simulink model "ddc_bpm_476_066"  (Simulink 7.8)
settings: Solver=ode45  StartTime=0.0  StopTime=2e-3  RelTol=1e-3
undefined symbols (not defined in the file): decim_factor_poly_35, dt_sim, frev_476, Fs_adc, n_ch, n_ovs, R_fofb, R_sec, R_sec_cfir, R_sec_pfir, xlipgetpartsetting
libraries: xbsIndex_r4 x1136, simulink x7
(part 1 of 10)
settings Model: Creator=lucas.russo  LastModifiedBy=lucas.russo
settings HardwareCC: ProdHWDeviceType=ASIC/FPGA->ASIC/FPGA  TargetIntDivRoundTo=Zero  TargetEndianess=LittleEndian  TargetHWDeviceType=MATLAB Host  ProdEqTarget=off

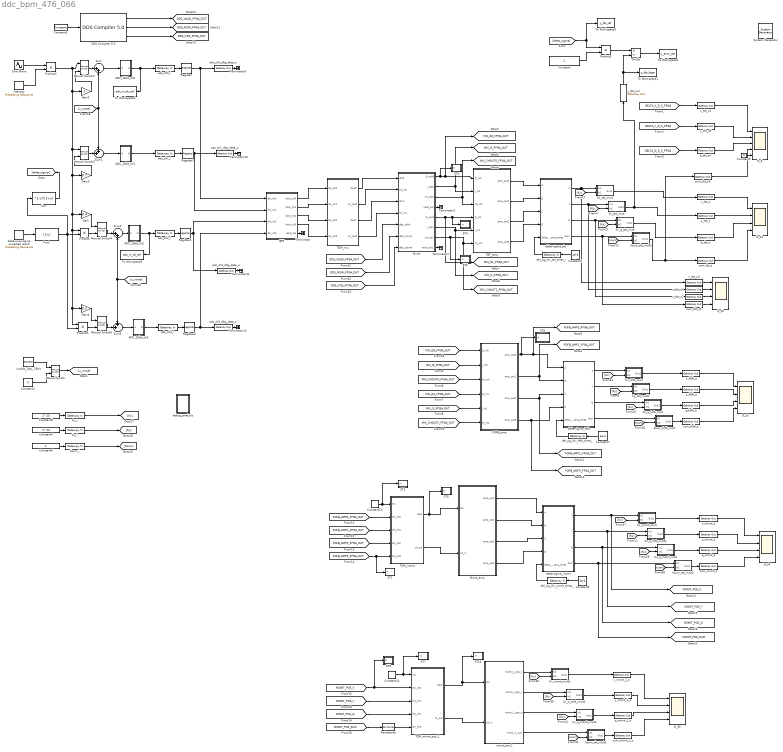
== system ddc_bpm_476_066 ==
  " System Generator" : xbsIndex_r4/ System Generator  Tag=genX  xilinxfamily=virtex6  part=xc6vlx240t  speed=-1  package=ff1156  synthesis_tool=XST  clock_wrapper=Clock Enables  directory=./netlist_ddc_bpm_476_066  proj_type=Project Navigator  Synth_file=XST Defaults  Impl_file=ISE Defaults  testbench=off  simulink_period=1/Fs_adc/n_ovs  sysclk_period=1/Fs_adc/n_ovs*1e9  dcm_input_clock_period=10  incr_netlist=off  trim_vbits=Everywhere in SubSystem  dbl_ovrd=According to Block Masks  core_generation=According to Block Masks  run_coregen=off  deprecated_control=off  eval_field=0  block_type=sysgen
  ADC_16bit_ch0 : Subsystem
  ADC_16bit_ch1 : Subsystem
  ADC_16bit_ch2 : Subsystem
  ADC_16bit_ch3 : Subsystem
  BPF : Subsystem
  Constant : Constant
  Constant1 : Constant  Value=1e-4  OutDataTypeStr=fixdt(1,26,22)
  Constant10 : xbsIndex_r4/Constant  const=0  gui_display_data_type=Boolean  arith_type=Boolean  n_bits=16  bin_pt=14  preci_type=Single  exp_width=8  frac_width=24  explicit_period=on  period=(1/Fs_adc*R_fofb)/n_ovs/2  equ=P=C  opselect=C  inp2=PCIN>>17  opr=+  inp1=P  carry=CIN  dbl_ovrd=off  block_type=constant
  Constant11 : xbsIndex_r4/Constant  const=0  gui_display_data_type=Boolean  arith_type=Boolean  n_bits=16  bin_pt=14  preci_type=Single  exp_width=8  frac_width=24  explicit_period=on  period=(1/Fs_adc*R_fofb*R_sec*R_sec_cfir*R_sec_pfir)/n_ovs/2  equ=P=C  opselect=C  inp2=PCIN>>17  opr=+  inp1=P  carry=CIN  dbl_ovrd=off  block_type=constant
  Constant2 : Constant  Value=0  SampleTime=0
  Constant3 : xbsIndex_r4/Constant  const=1  gui_display_data_type=Boolean  arith_type=Boolean  n_bits=24  bin_pt=22  preci_type=Single  exp_width=8  frac_width=24  explicit_period=on  period=dt_sim  equ=P=C  opselect=C  inp2=PCIN>>17  opr=+  inp1=P  carry=CIN  dbl_ovrd=off  block_type=constant
  Constant4 : Constant  Value=2^23
  Constant5 : Constant  Value=0
  Constant6 : Constant
  Constant7 : Constant  Value=1e-4  OutDataTypeStr=fixdt(1,26,22)
  Constant8 : Constant  Value=2^23
  Constant9 : Constant  Value=1e-4  OutDataTypeStr=fixdt(1,26,22)
  "DDS Compiler 5.0 " : xbsIndex_r4/DDS Compiler 5.0   partspresent=Phase_Generator_and_SIN_COS_LUT  dds_clock_rate=Fs_adc/1e6  channels=1  parameter_entry=Hardware_Parameters  spurious_free_dynamic_range=36  frequency_resolution=0.4  noise_shaping=Taylor_Series_Corrected  phase_width=30  output_width=24  output_selection=Sine_and_Cosine  negative_sine=on  negative_cosine=off  amplitude_mode=Unit_Circle  memory_type=Auto  optimization_goal=Auto  dsp48_use=Minimal  latency_configuration=Auto  latency=11  has_phase_out=off  has_aclken=off  has_aresetn=off  explicit_period=on  period=1/Fs_adc  data_has_tlast=Not_Required  has_tready=on  s_phase_has_tuser=Not_Required  m_data_has_tuser=Not_Required  m_phase_has_tuser=Not_Required  s_phase_tuser_width=1  s_config_sync_mode=On_Vector  phase_increment=Fixed  output_frequency1=0  output_frequency2=0  output_frequency3=0  output_frequency4=0  output_frequency5=0  output_frequency6=0  output_frequency7=0  output_frequency8=0  output_frequency9=0  output_frequency10=0  output_frequency11=0  output_frequency12=0  output_frequency13=0  output_frequency14=0  output_frequency15=0  output_frequency16=0  pinc1=dds_freq_bin  pinc2='0'  pinc3='0'  pinc4='0'  pinc5='0'  pinc6='0'  pinc7='0'  pinc8='0'  pinc9='0'  pinc10='0'  pinc11='0'  pinc12='0'  pinc13='0'  pinc14='0'  pinc15='0'  pinc16='0'  phase_offset=None  phase_offset_angles1=0  phase_offset_angles2=0  phase_offset_angles3=0  phase_offset_angles4=0  phase_offset_angles5=0  phase_offset_angles6=0  phase_offset_angles7=0  phase_offset_angles8=0  phase_offset_angles9=0  phase_offset_angles10=0  phase_offset_angles11=0  phase_offset_angles12=0  phase_offset_angles13=0  phase_offset_angles14=0  phase_offset_angles15=0  phase_offset_angles16=0  poff1='0'  poff2='0'  poff3='0'  poff4='0'  poff5='0'  poff6='0'  poff7='0'  poff8='0'  poff9='0'  poff10='0'  poff11='0'  poff12='0'  poff13='0'  poff14='0'  poff15='0'  poff16='0'  trim_axipin_name=on  por_mode=false  gui_behaviour=Sysgen  ip_name=DDS Compiler  ip_version=5.0  dsptool_ready=true  wrapper_available=true  port_translation_map={ 'aclken' => 'en', 'aresetn' => 'rst' }  ipcore_xco_need_fpga_part=true  ipcore_fpga_part=xlipgetpartsetting(gcb, {'virtex6', 'xc6vlx75t', '-3', 'ff784'})  ipcore_usecache=true  ipcore_useipmodelcache=true  ipcore_verbose=false  block_type=dds_compiler_v5_0
  D_S : Scope  NumInputPorts=5
      settings: TimeRange=0.0004  YMin=-1~0~10~0~0  YMax=1~0.00025~100~2.5~1  SaveName=ScopeData7  MaxDataPoints=1000000  SampleInput=on
  D_S{1..5} (5 alike) : Scope  NumInputPorts=4
      D_S1 settings: TimeRange=0.0003  YMin=-1~-1~-1~0.414326  YMax=1~1~1~0.414329  SaveName=ScopeData6  MaxDataPoints=1000000  SampleInput=on
      D_S2 settings: TimeRange=0.0003  YMin=-1~-1~0.95~0.81  YMax=1~1~1.05~0.84  MaxDataPoints=1000000  SampleInput=on
      D_S3 settings: TimeRange=0.0003  YMin=-1~-1~-1~0.0190031  YMax=1~1~1~0.0210035  SaveName=ScopeData2  MaxDataPoints=1000000  SampleInput=on
      D_S4 settings: TimeRange=0.0003  YMin=-1~-1~-1~0.0190031  YMax=1~1~1~0.0210035  SaveName=ScopeData3  MaxDataPoints=1000000  SampleInput=on
      D_S5 settings: TimeRange=0.0003  YMin=-1~-1~-1~0.0190031  YMax=1~1~1~0.0210035  SaveName=ScopeData20  MaxDataPoints=1000000  SampleInput=on
  Divide : Product  Inputs=*/
  FOFB_amp : Subsystem
  Fcn : Fcn  Expr=(1-u)/(1+u)
  Fcn1 : Fcn  Expr=(1-u)
  Gain : Gain  Gain=0.4
  Gain2 : Gain
  Gain3 : Gain  Gain=0.7
  Gain4 : Gain  Gain=0.1
  Ksum_fofb_mult : Subsystem
  Ksum_i : xbsIndex_r4/Gateway In  gui_display_data_type=Fixed-point  arith_type="Signed  (2's comp)"  n_bits=25  bin_pt=23  preci_type=Single  exp_width=8  frac_width=24  quantization=Truncate  overflow=Flag as error  period=1/Fs_adc  dbl_ovrd=off  timing_constraint=Data Rate  locs_specified=off  LOCs={}  inherit_from_input=off  UseAsADC=off  ADCChannel='1'  hdl_port=on  block_type=gatewayin
      settings: infoedit="Gateway in block.  Converts inputs of type Simulink integer, single, double and fixed point to  Xilinx fixed-point or floating-point data type.<br><br>Hardware notes:  In hardware these blocks become top level input ports."
  Ksum_tbt_mult1 : Subsystem
  Ksum_tbt_mult2 : Subsystem
  Ksum_tbt_mult3 : Subsystem
  Kx_fofb_mult : Subsystem
  Kx_i : xbsIndex_r4/Gateway In  gui_display_data_type=Fixed-point  arith_type="Signed  (2's comp)"  n_bits=25  bin_pt=0  preci_type=Single  exp_width=8  frac_width=24  quantization=Truncate  overflow=Flag as error  period=1/Fs_adc  dbl_ovrd=off  timing_constraint=Data Rate  locs_specified=off  LOCs={}  inherit_from_input=off  UseAsADC=off  ADCChannel='1'  hdl_port=on  block_type=gatewayin
      settings: infoedit="Gateway in block.  Converts inputs of type Simulink integer, single, double and fixed point to  Xilinx fixed-point or floating-point data type.<br><br>Hardware notes:  In hardware these blocks become top level input ports."
  Kx_monit_mult : Subsystem
  Kx_monit_mult1 : Subsystem
  Kx_q_fofb_mult : Subsystem
  Kx_q_fofb_mult1 : Subsystem
  Kx_q_fofb_mult2 : Subsystem
  Kx_q_monit_mult : Subsystem
  Kx_q_monit_mult1 : Subsystem
  Kx_q_tbt_mult : Subsystem
  Kx_tbt_mult : Subsystem
  Ky_i : xbsIndex_r4/Gateway In  gui_display_data_type=Fixed-point  arith_type="Signed  (2's comp)"  n_bits=25  bin_pt=0  preci_type=Single  exp_width=8  frac_width=24  quantization=Truncate  overflow=Flag as error  period=1/Fs_adc  dbl_ovrd=off  timing_constraint=Data Rate  locs_specified=off  LOCs={}  inherit_from_input=off  UseAsADC=off  ADCChannel='1'  hdl_port=on  block_type=gatewayin
      settings: infoedit="Gateway in block.  Converts inputs of type Simulink integer, single, double and fixed point to  Xilinx fixed-point or floating-point data type.<br><br>Hardware notes:  In hardware these blocks become top level input ports."
  Ky_tbt_mult : Subsystem
  Ky_tbt_mult1 : Subsystem
  Manual Switch : simulink/Signal Routing/Manual Switch  sw=0  action=0  varsize=off
  Manual Switch2 : simulink/Signal Routing/Manual Switch  sw=0  action=0  varsize=off
  Manual Switch3 : simulink/Signal Routing/Manual Switch  sw=0  action=0  varsize=off
  Manual Switch4 : simulink/Signal Routing/Manual Switch  sw=1  action=0  varsize=off
  Manual Switch5 : simulink/Signal Routing/Manual Switch  sw=1  action=0  varsize=off
  Mixer : Subsystem
  Monit_amp : Subsystem
  Product{,1..3} (4 alike) : Product  RndMeth=Zero
  Register{,1..3} (4 alike) : xbsIndex_r4/Register  init=0  rst=off  en=off  dbl_ovrd=off  block_type=register
  Reinterpret : xbsIndex_r4/Reinterpret  force_arith_type=on  arith_type="Signed  (2's comp)"  force_bin_pt=on  bin_pt=24  block_type=reinterpret
  ST1 : Subsystem
  ST10 : Subsystem
  ST2 : Subsystem
  ST3 : Subsystem
  ST4 : Subsystem
  ST5 : Subsystem
  ST6 : Subsystem
  ST7 : Subsystem
  ST8 : Subsystem
  ST9 : Subsystem
  Sine Wave : Sin  Frequency=2*pi*frev_476  SampleTime=0
  Sum : Sum  Inputs=|++
  Sum1 : Sum  Inputs=++|
  Sum2 : Sum  Inputs=|++
  Sum3 : Sum  Inputs=++|
  TBT_amp : Subsystem
  TDM_mix : Subsystem
  TDM_monit : Subsystem
  TDM_monit_pos_1 : Subsystem
  Terminator{,1,4,9..12} (7 alike) : Terminator
  To Workspace1 : ToWorkspace  VariableName=y_tbt_fpga  SampleTime=-1  SaveFormat=Structure With Time
  To Workspace2 : ToWorkspace  VariableName=y_error_tbt  SampleTime=-1  SaveFormat=Structure With Time
  To Workspace3 : ToWorkspace  VariableName=y_tbt_ref  SampleTime=-1  SaveFormat=Structure With Time
  To Workspace4 : ToWorkspace  VariableName=adc_in_ab_ref  SampleTime=-1  SaveFormat=Structure With Time
  To Workspace5 : ToWorkspace  VariableName=adc_in_cd_ref  SampleTime=-1  SaveFormat=Structure With Time
  adc_ch0_dbg_data_o : xbsIndex_r4/Gateway Out  inherit_from_input=on  hdl_port=on  timing_constraint=Data Rate  locs_specified=off  LOCs={}  UseAsDAC=off  DACChannel='1'  block_type=gatewayout
      settings: infoedit="Gateway out block.  Converts Xilinx fixed-point or floating-point type inputs into ouputs of type Simulink integer, single, double, or fixed point.<br><br>Hardware notes:  In hardware these blocks become top level output ports or are discarded, depending on how they are configured."
  adc_ch0_i : xbsIndex_r4/Gateway In  gui_display_data_type=Fixed-point  arith_type="Signed  (2's comp)"  n_bits=16  bin_pt=15  preci_type=Single  exp_width=8  frac_width=24  quantization=Truncate  overflow=Flag as error  period=1/Fs_adc  dbl_ovrd=off  timing_constraint=None  locs_specified=off  LOCs={}  inherit_from_input=off  UseAsADC=off  ADCChannel='1'  hdl_port=on  block_type=gatewayin
      settings: infoedit="Gateway in block.  Converts inputs of type Simulink integer, single, double and fixed point to  Xilinx fixed-point or floating-point data type.<br><br>Hardware notes:  In hardware these blocks become top level input ports."
  adc_ch1_dbg_data_o : xbsIndex_r4/Gateway Out  inherit_from_input=on  hdl_port=on  timing_constraint=Data Rate  locs_specified=off  LOCs={}  UseAsDAC=off  DACChannel='1'  block_type=gatewayout
      settings: infoedit="Gateway out block.  Converts Xilinx fixed-point or floating-point type inputs into ouputs of type Simulink integer, single, double, or fixed point.<br><br>Hardware notes:  In hardware these blocks become top level output ports or are discarded, depending on how they are configured."
  adc_ch1_i : xbsIndex_r4/Gateway In  gui_display_data_type=Fixed-point  arith_type="Signed  (2's comp)"  n_bits=16  bin_pt=15  preci_type=Single  exp_width=8  frac_width=24  quantization=Truncate  overflow=Flag as error  period=1/Fs_adc  dbl_ovrd=off  timing_constraint=None  locs_specified=off  LOCs={}  inherit_from_input=off  UseAsADC=off  ADCChannel='1'  hdl_port=on  block_type=gatewayin
      settings: infoedit="Gateway in block.  Converts inputs of type Simulink integer, single, double and fixed point to  Xilinx fixed-point or floating-point data type.<br><br>Hardware notes:  In hardware these blocks become top level input ports."
  adc_ch2_dbg_data_o : xbsIndex_r4/Gateway Out  inherit_from_input=on  hdl_port=on  timing_constraint=Data Rate  locs_specified=off  LOCs={}  UseAsDAC=off  DACChannel='1'  block_type=gatewayout
      settings: infoedit="Gateway out block.  Converts Xilinx fixed-point or floating-point type inputs into ouputs of type Simulink integer, single, double, or fixed point.<br><br>Hardware notes:  In hardware these blocks become top level output ports or are discarded, depending on how they are configured."
  adc_ch2_i : xbsIndex_r4/Gateway In  gui_display_data_type=Fixed-point  arith_type="Signed  (2's comp)"  n_bits=16  bin_pt=15  preci_type=Single  exp_width=8  frac_width=24  quantization=Truncate  overflow=Flag as error  period=1/Fs_adc  dbl_ovrd=off  timing_constraint=None  locs_specified=off  LOCs={}  inherit_from_input=off  UseAsADC=off  ADCChannel='1'  hdl_port=on  block_type=gatewayin
      settings: infoedit="Gateway in block.  Converts inputs of type Simulink integer, single, double and fixed point to  Xilinx fixed-point or floating-point data type.<br><br>Hardware notes:  In hardware these blocks become top level input ports."
  adc_ch3_dbg_data_o : xbsIndex_r4/Gateway Out  inherit_from_input=on  hdl_port=on  timing_constraint=Data Rate  locs_specified=off  LOCs={}  UseAsDAC=off  DACChannel='1'  block_type=gatewayout
      settings: infoedit="Gateway out block.  Converts Xilinx fixed-point or floating-point type inputs into ouputs of type Simulink integer, single, double, or fixed point.<br><br>Hardware notes:  In hardware these blocks become top level output ports or are discarded, depending on how they are configured."
  adc_ch3_i : xbsIndex_r4/Gateway In  gui_display_data_type=Fixed-point  arith_type="Signed  (2's comp)"  n_bits=16  bin_pt=15  preci_type=Single  exp_width=8  frac_width=24  quantization=Truncate  overflow=Flag as error  period=1/Fs_adc  dbl_ovrd=off  timing_constraint=None  locs_specified=off  LOCs={}  inherit_from_input=off  UseAsADC=off  ADCChannel='1'  hdl_port=on  block_type=gatewayin
      settings: infoedit="Gateway in block.  Converts inputs of type Simulink integer, single, double and fixed point to  Xilinx fixed-point or floating-point data type.<br><br>Hardware notes:  In hardware these blocks become top level input ports."
  debug_analysis : Subsystem
  del_sig_div_fofb_thres_i : xbsIndex_r4/Gateway In  gui_display_data_type=Fixed-point  arith_type="Signed  (2's comp)"  n_bits=26  bin_pt=22  preci_type=Single  exp_width=8  frac_width=24  quantization=Truncate  overflow=Flag as error  period=1/Fs_adc  dbl_ovrd=off  timing_constraint=Data Rate  locs_specified=off  LOCs={}  inherit_from_input=off  UseAsADC=off  ADCChannel='1'  hdl_port=on  block_type=gatewayin
      settings: infoedit="Gateway in block.  Converts inputs of type Simulink integer, single, double and fixed point to  Xilinx fixed-point or floating-point data type.<br><br>Hardware notes:  In hardware these blocks become top level input ports."
  del_sig_div_monit_thres_i : xbsIndex_r4/Gateway In  gui_display_data_type=Fixed-point  arith_type="Signed  (2's comp)"  n_bits=26  bin_pt=22  preci_type=Single  exp_width=8  frac_width=24  quantization=Truncate  overflow=Flag as error  period=1/Fs_adc  dbl_ovrd=off  timing_constraint=Data Rate  locs_specified=off  LOCs={}  inherit_from_input=off  UseAsADC=off  ADCChannel='1'  hdl_port=on  block_type=gatewayin
      settings: infoedit="Gateway in block.  Converts inputs of type Simulink integer, single, double and fixed point to  Xilinx fixed-point or floating-point data type.<br><br>Hardware notes:  In hardware these blocks become top level input ports."
  del_sig_div_tbt_thres_i : xbsIndex_r4/Gateway In  gui_display_data_type=Fixed-point  arith_type="Signed  (2's comp)"  n_bits=26  bin_pt=22  preci_type=Single  exp_width=8  frac_width=24  quantization=Truncate  overflow=Flag as error  period=1/Fs_adc  dbl_ovrd=off  timing_constraint=Data Rate  locs_specified=off  LOCs={}  inherit_from_input=off  UseAsADC=off  ADCChannel='1'  hdl_port=on  block_type=gatewayin
      settings: infoedit="Gateway in block.  Converts inputs of type Simulink integer, single, double and fixed point to  Xilinx fixed-point or floating-point data type.<br><br>Hardware notes:  In hardware these blocks become top level input ports."
  delta-over-sigma expected result : simulink/Sources/Repeating Sequence  rep_seq_t=[0 0.25e-4 0.25e-4 0.5e-4 0.5e-4 0.75e-4 0.75e-4 1e-4]  rep_seq_y=0.5 * [1 1 1 1 1 1 1 1]
  delta-sigma_fofb : Subsystem
  delta-sigma_monit : Subsystem
  delta-sigma_tbt : Subsystem
  intensity : simulink/Sources/Repeating Sequence  rep_seq_t=[0 1e-4 1e-4 2e-4 2e-4 3e-4 3e-4 4e-4]  rep_seq_y=[1 1 0.1 0.1 0.01 0.01 0.001 0.001]
  monit_pos_1 : Subsystem
  q_fofb_o : xbsIndex_r4/Gateway Out  inherit_from_input=on  hdl_port=on  timing_constraint=None  locs_specified=off  LOCs={}  UseAsDAC=off  DACChannel='1'  block_type=gatewayout
      settings: infoedit="Gateway out block.  Converts Xilinx fixed-point or floating-point type inputs into ouputs of type Simulink integer, single, double, or fixed point.<br><br>Hardware notes:  In hardware these blocks become top level output ports or are discarded, depending on how they are configured."
  q_monit_1_o : xbsIndex_r4/Gateway Out  inherit_from_input=on  hdl_port=on  timing_constraint=None  locs_specified=off  LOCs={}  UseAsDAC=off  DACChannel='1'  block_type=gatewayout
      settings: infoedit="Gateway out block.  Converts Xilinx fixed-point or floating-point type inputs into ouputs of type Simulink integer, single, double, or fixed point.<br><br>Hardware notes:  In hardware these blocks become top level output ports or are discarded, depending on how they are configured."
  q_monit_o : xbsIndex_r4/Gateway Out  inherit_from_input=on  hdl_port=on  timing_constraint=None  locs_specified=off  LOCs={}  UseAsDAC=off  DACChannel='1'  block_type=gatewayout
      settings: infoedit="Gateway out block.  Converts Xilinx fixed-point or floating-point type inputs into ouputs of type Simulink integer, single, double, or fixed point.<br><br>Hardware notes:  In hardware these blocks become top level output ports or are discarded, depending on how they are configured."
  q_tbt_o : xbsIndex_r4/Gateway Out  inherit_from_input=on  hdl_port=on  timing_constraint=Data Rate  locs_specified=off  LOCs={}  UseAsDAC=off  DACChannel='1'  block_type=gatewayout
      settings: infoedit="Gateway out block.  Converts Xilinx fixed-point or floating-point type inputs into ouputs of type Simulink integer, single, double, or fixed point.<br><br>Hardware notes:  In hardware these blocks become top level output ports or are discarded, depending on how they are configured."
  q_tbt_o4 : xbsIndex_r4/Gateway Out  inherit_from_input=on  hdl_port=off  timing_constraint=None  locs_specified=off  LOCs={}  UseAsDAC=off  DACChannel='1'  block_type=gatewayout
      settings: infoedit="Gateway out block.  Converts Xilinx fixed-point or floating-point type inputs into ouputs of type Simulink integer, single, double, or fixed point.<br><br>Hardware notes:  In hardware these blocks become top level output ports or are discarded, depending on how they are configured."
  sum_fofb_o : xbsIndex_r4/Gateway Out  inherit_from_input=on  hdl_port=on  timing_constraint=None  locs_specified=off  LOCs={}  UseAsDAC=off  DACChannel='1'  block_type=gatewayout
      settings: infoedit="Gateway out block.  Converts Xilinx fixed-point or floating-point type inputs into ouputs of type Simulink integer, single, double, or fixed point.<br><br>Hardware notes:  In hardware these blocks become top level output ports or are discarded, depending on how they are configured."
  sum_monit_1_o : xbsIndex_r4/Gateway Out  inherit_from_input=on  hdl_port=on  timing_constraint=None  locs_specified=off  LOCs={}  UseAsDAC=off  DACChannel='1'  block_type=gatewayout
      settings: infoedit="Gateway out block.  Converts Xilinx fixed-point or floating-point type inputs into ouputs of type Simulink integer, single, double, or fixed point.<br><br>Hardware notes:  In hardware these blocks become top level output ports or are discarded, depending on how they are configured."
  sum_monit_o : xbsIndex_r4/Gateway Out  inherit_from_input=on  hdl_port=on  timing_constraint=None  locs_specified=off  LOCs={}  UseAsDAC=off  DACChannel='1'  block_type=gatewayout
      settings: infoedit="Gateway out block.  Converts Xilinx fixed-point or floating-point type inputs into ouputs of type Simulink integer, single, double, or fixed point.<br><br>Hardware notes:  In hardware these blocks become top level output ports or are discarded, depending on how they are configured."
  sum_tbt_o : xbsIndex_r4/Gateway Out  inherit_from_input=on  hdl_port=on  timing_constraint=Data Rate  locs_specified=off  LOCs={}  UseAsDAC=off  DACChannel='1'  block_type=gatewayout
      settings: infoedit="Gateway out block.  Converts Xilinx fixed-point or floating-point type inputs into ouputs of type Simulink integer, single, double, or fixed point.<br><br>Hardware notes:  In hardware these blocks become top level output ports or are discarded, depending on how they are configured."
  sum_tbt_o1 : xbsIndex_r4/Gateway Out  inherit_from_input=on  hdl_port=off  timing_constraint=Data Rate  locs_specified=off  LOCs={}  UseAsDAC=off  DACChannel='1'  block_type=gatewayout
      settings: infoedit="Gateway out block.  Converts Xilinx fixed-point or floating-point type inputs into ouputs of type Simulink integer, single, double, or fixed point.<br><br>Hardware notes:  In hardware these blocks become top level output ports or are discarded, depending on how they are configured."
  sum_tbt_o5 : xbsIndex_r4/Gateway Out  inherit_from_input=on  hdl_port=off  timing_constraint=None  locs_specified=off  LOCs={}  UseAsDAC=off  DACChannel='1'  block_type=gatewayout
      settings: infoedit="Gateway out block.  Converts Xilinx fixed-point or floating-point type inputs into ouputs of type Simulink integer, single, double, or fixed point.<br><br>Hardware notes:  In hardware these blocks become top level output ports or are discarded, depending on how they are configured."
  unoise_1lsb_ 16bit : UniformRandomNumber  Minimum=-0.5*(2/2^16)  Maximum=0.5*(2/2^16)  Seed=49728613  SampleTime=0
  x_fofb_o : xbsIndex_r4/Gateway Out  inherit_from_input=on  hdl_port=on  timing_constraint=None  locs_specified=off  LOCs={}  UseAsDAC=off  DACChannel='1'  block_type=gatewayout
      settings: infoedit="Gateway out block.  Converts Xilinx fixed-point or floating-point type inputs into ouputs of type Simulink integer, single, double, or fixed point.<br><br>Hardware notes:  In hardware these blocks become top level output ports or are discarded, depending on how they are configured."
  x_monit_1_o : xbsIndex_r4/Gateway Out  inherit_from_input=on  hdl_port=on  timing_constraint=None  locs_specified=off  LOCs={}  UseAsDAC=off  DACChannel='1'  block_type=gatewayout
      settings: infoedit="Gateway out block.  Converts Xilinx fixed-point or floating-point type inputs into ouputs of type Simulink integer, single, double, or fixed point.<br><br>Hardware notes:  In hardware these blocks become top level output ports or are discarded, depending on how they are configured."
  x_monit_o : xbsIndex_r4/Gateway Out  inherit_from_input=on  hdl_port=on  timing_constraint=None  locs_specified=off  LOCs={}  UseAsDAC=off  DACChannel='1'  block_type=gatewayout
      settings: infoedit="Gateway out block.  Converts Xilinx fixed-point or floating-point type inputs into ouputs of type Simulink integer, single, double, or fixed point.<br><br>Hardware notes:  In hardware these blocks become top level output ports or are discarded, depending on how they are configured."
  x_tbt_o : xbsIndex_r4/Gateway Out  inherit_from_input=on  hdl_port=on  timing_constraint=Data Rate  locs_specified=off  LOCs={}  UseAsDAC=off  DACChannel='1'  block_type=gatewayout
      settings: infoedit="Gateway out block.  Converts Xilinx fixed-point or floating-point type inputs into ouputs of type Simulink integer, single, double, or fixed point.<br><br>Hardware notes:  In hardware these blocks become top level output ports or are discarded, depending on how they are configured."
  x_tbt_o1 : xbsIndex_r4/Gateway Out  inherit_from_input=on  hdl_port=off  timing_constraint=None  locs_specified=off  LOCs={}  UseAsDAC=off  DACChannel='1'  block_type=gatewayout
      settings: infoedit="Gateway out block.  Converts Xilinx fixed-point or floating-point type inputs into ouputs of type Simulink integer, single, double, or fixed point.<br><br>Hardware notes:  In hardware these blocks become top level output ports or are discarded, depending on how they are configured."
  x_tbt_o2 : xbsIndex_r4/Gateway Out  inherit_from_input=on  hdl_port=off  timing_constraint=Data Rate  locs_specified=off  LOCs={}  UseAsDAC=off  DACChannel='1'  block_type=gatewayout
      settings: infoedit="Gateway out block.  Converts Xilinx fixed-point or floating-point type inputs into ouputs of type Simulink integer, single, double, or fixed point.<br><br>Hardware notes:  In hardware these blocks become top level output ports or are discarded, depending on how they are configured."
  y_fofb_o : xbsIndex_r4/Gateway Out  inherit_from_input=on  hdl_port=on  timing_constraint=None  locs_specified=off  LOCs={}  UseAsDAC=off  DACChannel='1'  block_type=gatewayout
      settings: infoedit="Gateway out block.  Converts Xilinx fixed-point or floating-point type inputs into ouputs of type Simulink integer, single, double, or fixed point.<br><br>Hardware notes:  In hardware these blocks become top level output ports or are discarded, depending on how they are configured."
  y_monit_1_o : xbsIndex_r4/Gateway Out  inherit_from_input=on  hdl_port=on  timing_constraint=None  locs_specified=off  LOCs={}  UseAsDAC=off  DACChannel='1'  block_type=gatewayout
      settings: infoedit="Gateway out block.  Converts Xilinx fixed-point or floating-point type inputs into ouputs of type Simulink integer, single, double, or fixed point.<br><br>Hardware notes:  In hardware these blocks become top level output ports or are discarded, depending on how they are configured."
  y_monit_o : xbsIndex_r4/Gateway Out  inherit_from_input=on  hdl_port=on  timing_constraint=None  locs_specified=off  LOCs={}  UseAsDAC=off  DACChannel='1'  block_type=gatewayout
      settings: infoedit="Gateway out block.  Converts Xilinx fixed-point or floating-point type inputs into ouputs of type Simulink integer, single, double, or fixed point.<br><br>Hardware notes:  In hardware these blocks become top level output ports or are discarded, depending on how they are configured."
  y_tbt_o : xbsIndex_r4/Gateway Out  inherit_from_input=on  hdl_port=on  timing_constraint=Data Rate  locs_specified=off  LOCs={}  UseAsDAC=off  DACChannel='1'  block_type=gatewayout
      settings: infoedit="Gateway out block.  Converts Xilinx fixed-point or floating-point type inputs into ouputs of type Simulink integer, single, double, or fixed point.<br><br>Hardware notes:  In hardware these blocks become top level output ports or are discarded, depending on how they are configured."
  y_tbt_o1 : xbsIndex_r4/Gateway Out  inherit_from_input=on  hdl_port=off  timing_constraint=Data Rate  locs_specified=off  LOCs={}  UseAsDAC=off  DACChannel='1'  block_type=gatewayout
      settings: infoedit="Gateway out block.  Converts Xilinx fixed-point or floating-point type inputs into ouputs of type Simulink integer, single, double, or fixed point.<br><br>Hardware notes:  In hardware these blocks become top level output ports or are discarded, depending on how they are configured."
  y_tbt_o2 : xbsIndex_r4/Gateway Out  inherit_from_input=on  hdl_port=off  timing_constraint=Data Rate  locs_specified=off  LOCs={}  UseAsDAC=off  DACChannel='1'  block_type=gatewayout
      settings: infoedit="Gateway out block.  Converts Xilinx fixed-point or floating-point type inputs into ouputs of type Simulink integer, single, double, or fixed point.<br><br>Hardware notes:  In hardware these blocks become top level output ports or are discarded, depending on how they are configured."
  y_tbt_o6 : xbsIndex_r4/Gateway Out  inherit_from_input=on  hdl_port=off  timing_constraint=None  locs_specified=off  LOCs={}  UseAsDAC=off  DACChannel='1'  block_type=gatewayout
      settings: infoedit="Gateway out block.  Converts Xilinx fixed-point or floating-point type inputs into ouputs of type Simulink integer, single, double, or fixed point.<br><br>Hardware notes:  In hardware these blocks become top level output ports or are discarded, depending on how they are configured."
  y_tbt_out : xbsIndex_r4/Gateway Out  inherit_from_input=on  hdl_port=off  timing_constraint=None  locs_specified=off  LOCs={}  UseAsDAC=off  DACChannel='1'  block_type=gatewayout
      settings: infoedit="Gateway out block.  Converts Xilinx fixed-point or floating-point type inputs into ouputs of type Simulink integer, single, double, or fixed point.<br><br>Hardware notes:  In hardware these blocks become top level output ports or are discarded, depending on how they are configured."
  tag scope: DDS_COS_FPGA_OUT=global, DDS_MSIN_FPGA_OUT=global, DDS_VALID_FPGA_OUT=global, FOFB_AMP0_FPGA_OUT=global, FOFB_AMP1_FPGA_OUT=global, FOFB_AMP2_FPGA_OUT=global, FOFB_AMP3_FPGA_OUT=global, MIX_CHOUT0_FPGA_OUT=global, MIX_CHOUT1_FPGA_OUT=global, MIX_I0_FPGA_OUT=global, MIX_I1_FPGA_OUT=global, MIX_Q0_FPGA_OUT=global, MIX_Q1_FPGA_OUT=global, MONIT_POS_Q=global, MONIT_POS_SUM=global, MONIT_POS_X=global, MONIT_POS_Y=global
  wires:
  delta-over-sigma expected result/1 -> Fcn1/1
  Fcn/1 -> [delta_sigma]
  ADC_16bit_ch0/1(D) -> To Workspace4/1, adc_ch0_i/1
  Constant3/1 -> "DDS Compiler 5.0 "/1
  "DDS Compiler 5.0 "/1 -> [DDS_VALID_FPGA_OUT]
  "DDS Compiler 5.0 "/2 -> [DDS_MSIN_FPGA_OUT]
  "DDS Compiler 5.0 "/3 -> [DDS_COS_FPGA_OUT]
  ADC_16bit_ch1/1(D) -> adc_ch1_i/1
  ADC_16bit_ch2/1(D) -> To Workspace5/1, adc_ch2_i/1
  ADC_16bit_ch3/1(D) -> adc_ch3_i/1
  Constant/1 -> Product3/2
  Product3/1 -> Divide/1
  Divide/1 -> To Workspace2/1
  [delta_sigma] -> Product3/1, To Workspace3/1
  [DELTA_X_D_S_FPGA] -> x_tbt_o1/1
  [DELTA_Y_D_S_FPGA] -> y_tbt_o6/1
  [DELTA_Q_D_S_FPGA] -> q_tbt_o4/1
  x_tbt_o1/1 -> D_S/1
  y_tbt_o6/1 -> D_S/2
  q_tbt_o4/1 -> D_S/3
  sum_tbt_o5/1 -> D_S/4
  x_tbt_o/1 -> D_S1/1
  y_tbt_o/1 -> D_S1/2
  q_tbt_o/1 -> D_S1/3
  sum_tbt_o/1 -> D_S1/4
  y_tbt_out/1 -> Divide/2, To Workspace1/1
  del_sig_div_tbt_thres_i/1 -> delta-sigma_tbt/5(Delta_sigma_thres)
  Fcn1/1 -> Product/2, Product1/2, Fcn/1
  Constant1/1 -> del_sig_div_tbt_thres_i/1
  intensity/1 -> Product2/2
  Sine Wave/1 -> Product2/1
  Product2/1 -> Manual Switch2/1, Gain2/1, Manual Switch3/1, Gain3/1, Product/1, Product1/1, Gain4/1, Gain/1
  Sum/1 -> ADC_16bit_ch0/1(A)
  Sum1/1 -> ADC_16bit_ch1/1(A)
  Sum2/1 -> ADC_16bit_ch2/1(A)
  Sum3/1 -> ADC_16bit_ch3/1(A)
  unoise_1lsb_ 16bit/1 -> Manual Switch/1
  Constant2/1 -> Manual Switch/2
  Manual Switch/1 -> [u_noise]
  [u_noise] -> Sum/2, Sum1/1
  [u_noise] -> Sum2/2, Sum3/1
  Constant5/1 -> D_S/5
  delta-sigma_tbt/1(X) -> Kx_tbt_mult/1(In1), x_tbt_o2/1
  delta-sigma_tbt/3(Q) -> Kx_q_tbt_mult/1(In1), y_tbt_o2/1
  [Kx] -> Kx_tbt_mult/2(In2)
  [Kx] -> Kx_q_tbt_mult/2(In2)
  delta-sigma_tbt/4(Sum) -> Ksum_tbt_mult3/1(In1), sum_tbt_o1/1
  Ksum_tbt_mult3/1(Out1) -> sum_tbt_o/1, sum_tbt_o5/1
  [Ksum] -> Ksum_tbt_mult3/2(In2)
  Constant6/1 -> Ksum_i/1
  Constant8/1 -> Kx_i/1
  Constant4/1 -> Ky_i/1
  Kx_i/1 -> [Kx]
  Ky_i/1 -> [Ky]
  Ksum_i/1 -> [Ksum]
  adc_ch0_i/1 -> Register/1
  adc_ch1_i/1 -> Register1/1
  adc_ch2_i/1 -> Register2/1
  adc_ch3_i/1 -> Register3/1
  [DDS_VALID_FPGA_OUT] -> Mixer/5(dds_valid)
  [DDS_COS_FPGA_OUT] -> Mixer/7(dds_cosine)
  [DDS_MSIN_FPGA_OUT] -> Mixer/6(dds_msine)
  adc_ch0_dbg_data_o/1 -> Terminator9/1
  adc_ch1_dbg_data_o/1 -> Terminator10/1
  adc_ch2_dbg_data_o/1 -> Terminator11/1
  adc_ch3_dbg_data_o/1 -> Terminator12/1
  TDM_mix/2(ch_out0) -> Mixer/2(ch_in0)
  TDM_mix/3(dout1) -> Mixer/3(din1)
  TDM_mix/4(ch_out1) -> Mixer/4(ch_in1)
  BPF/1(dout_ch0) -> TDM_mix/1(din_ch0)
  BPF/2(dout_ch1) -> TDM_mix/2(din_ch1)
  BPF/3(dout_ch2) -> TDM_mix/3(din_ch2)
  BPF/4(dout_ch3) -> TDM_mix/4(din_ch3)
  TDM_mix/1(dout0) -> Mixer/1(din0)
  Mixer/1(Q_out0) -> [MIX_Q0_FPGA_OUT], TBT_amp/1(Q_in0), ST3/1(In)
  Mixer/2(I_out0) -> TBT_amp/2(I_in0), [MIX_I0_FPGA_OUT]
  Mixer/3(ch_out0) -> TBT_amp/3(ch_in0), [MIX_CHOUT0_FPGA_OUT]
  Mixer/5(Q_out1) -> [MIX_Q1_FPGA_OUT], TBT_amp/4(Q_in1), ST4/1(In)
  Mixer/6(I_out1) -> TBT_amp/5(I_in1), [MIX_I1_FPGA_OUT]
  Mixer/7(ch_out1) -> TBT_amp/6(ch_in1), [MIX_CHOUT1_FPGA_OUT], ST6/1(In)
  BPF/5(valid_out) -> Terminator/1
  Mixer/4(valid_out) -> Terminator1/1
  Mixer/8(valid_out1) -> Terminator4/1
  TBT_amp/1(amp_out0) -> delta-sigma_tbt/1(A)
  TBT_amp/2(amp_out1) -> delta-sigma_tbt/2(B)
  TBT_amp/3(amp_out2) -> delta-sigma_tbt/3(C)
  TBT_amp/4(amp_out3) -> delta-sigma_tbt/4(D)
  delta-sigma_tbt/2(Y) -> y_tbt_o1/1, Ky_tbt_mult/1(In1)
  y_tbt_o1/1 -> D_S2/2
  x_tbt_o2/1 -> D_S2/1
  y_tbt_o2/1 -> D_S2/3
  sum_tbt_o1/1 -> D_S2/4
  del_sig_div_fofb_thres_i/1 -> delta-sigma_fofb/5(Delta_sigma_thres)
  Constant7/1 -> del_sig_div_fofb_thres_i/1
  x_fofb_o/1 -> D_S3/1
  y_fofb_o/1 -> D_S3/2
  q_fofb_o/1 -> D_S3/3
  sum_fofb_o/1 -> D_S3/4
  [Kx] -> Kx_fofb_mult/2(In2)
  [Kx] -> Kx_q_fofb_mult/2(In2)
  [Ksum] -> Ksum_fofb_mult/2(In2)
  delta-sigma_fofb/1(X) -> Kx_fofb_mult/1(In1)
  Kx_fofb_mult/1(Out1) -> x_fofb_o/1
  delta-sigma_fofb/3(Q) -> Kx_q_fofb_mult/1(In1)
  Kx_q_fofb_mult/1(Out1) -> q_fofb_o/1
  delta-sigma_fofb/4(Sum) -> Ksum_fofb_mult/1(In1)
  Ksum_fofb_mult/1(Out1) -> sum_fofb_o/1
  [Ky] -> Ky_tbt_mult1/2(In2)
  delta-sigma_fofb/2(Y) -> Ky_tbt_mult1/1(In1)
  Ky_tbt_mult1/1(Out1) -> y_fofb_o/1
  FOFB_amp/1(amp_out0) -> delta-sigma_fofb/1(A), [FOFB_AMP0_FPGA_OUT], ST8/1(In)
  FOFB_amp/2(amp_out1) -> delta-sigma_fofb/2(B), [FOFB_AMP1_FPGA_OUT]
  FOFB_amp/3(amp_out2) -> delta-sigma_fofb/3(C), [FOFB_AMP2_FPGA_OUT]
  FOFB_amp/4(amp_out3) -> delta-sigma_fofb/4(D), [FOFB_AMP3_FPGA_OUT]
  [MIX_Q0_FPGA_OUT] -> FOFB_amp/1(Q_in0)
  [MIX_I0_FPGA_OUT] -> FOFB_amp/2(I_in0)
  [MIX_CHOUT0_FPGA_OUT] -> FOFB_amp/3(ch_in0)
  [MIX_Q1_FPGA_OUT] -> FOFB_amp/4(Q_in1)
  [MIX_I1_FPGA_OUT] -> FOFB_amp/5(I_in1)
  [MIX_CHOUT1_FPGA_OUT] -> FOFB_amp/6(ch_in1)
  x_monit_o/1 -> D_S4/1
  sum_monit_o/1 -> D_S4/4
  y_monit_o/1 -> D_S4/2
  q_monit_o/1 -> D_S4/3
  [Kx] -> Kx_monit_mult/2(In2)
  [Kx] -> Kx_q_monit_mult/2(In2)
  [Ksum] -> Ksum_tbt_mult2/2(In2)
  Kx_monit_mult/1(Out1) -> x_monit_o/1
  Kx_q_monit_mult/1(Out1) -> q_monit_o/1
  Ksum_tbt_mult2/1(Out1) -> sum_monit_o/1
  Monit_amp/1(amp_out0) -> delta-sigma_monit/1(A)
  Monit_amp/2(amp_out1) -> delta-sigma_monit/2(B)
  Monit_amp/3(amp_out2) -> delta-sigma_monit/3(C)
  Monit_amp/4(amp_out3) -> delta-sigma_monit/4(D)
  Constant10/1 -> ST1/1(In), TDM_monit/1(rst)
  [FOFB_AMP0_FPGA_OUT] -> TDM_monit/2(din_ch0)
  [FOFB_AMP1_FPGA_OUT] -> TDM_monit/3(din_ch1)
  [FOFB_AMP2_FPGA_OUT] -> TDM_monit/4(din_ch2)
  [FOFB_AMP3_FPGA_OUT] -> ST2/1(In), TDM_monit/5(din_ch3)
  [Ky] -> Kx_q_fofb_mult1/2(In2)
  Kx_q_fofb_mult1/1(Out1) -> y_monit_o/1
  Constant9/1 -> del_sig_div_monit_thres_i/1
  delta-sigma_monit/4(Sum) -> Ksum_tbt_mult2/1(In1), [MONIT_POS_SUM]
  delta-sigma_monit/3(Q) -> Kx_q_monit_mult/1(In1), [MONIT_POS_Q]
  delta-sigma_monit/2(Y) -> Kx_q_fofb_mult1/1(In1), [MONIT_POS_Y]
  delta-sigma_monit/1(X) -> Kx_monit_mult/1(In1), [MONIT_POS_X]
  del_sig_div_monit_thres_i/1 -> delta-sigma_monit/5(Delta_sigma_thres)
  TDM_monit/1(dout) -> Monit_amp/1(din), ST5/1(In)
  TDM_monit/2(ch_out) -> Monit_amp/2(ch_in)
  [Ky] -> Ky_tbt_mult/2(In2)
  Ky_tbt_mult/1(Out1) -> y_tbt_o/1, y_tbt_out/1
  Kx_tbt_mult/1(Out1) -> x_tbt_o/1
  Kx_q_tbt_mult/1(Out1) -> q_tbt_o/1
  Register/1 -> adc_ch0_dbg_data_o/1, BPF/1(din_ch0)
  Register1/1 -> adc_ch1_dbg_data_o/1, BPF/2(din_ch1)
  Register2/1 -> adc_ch2_dbg_data_o/1, BPF/3(din_ch2)
  Register3/1 -> adc_ch3_dbg_data_o/1, BPF/4(din_ch3)
  Manual Switch2/1 -> Sum/1
  Gain2/1 -> Manual Switch2/2
  Manual Switch3/1 -> Sum1/2
  Gain3/1 -> Manual Switch3/2
  Gain/1 -> Manual Switch4/1
  Product/1 -> Manual Switch4/2
  Manual Switch4/1 -> Sum2/1
  Gain4/1 -> Manual Switch5/1
  Manual Switch5/1 -> Sum3/2
  Product1/1 -> Manual Switch5/2
  x_monit_1_o/1 -> D_S5/1
  sum_monit_1_o/1 -> D_S5/4
  y_monit_1_o/1 -> D_S5/2
  q_monit_1_o/1 -> D_S5/3
  [MONIT_POS_Y] -> TDM_monit_pos_1/3(din_ch1)
  [MONIT_POS_X] -> TDM_monit_pos_1/2(din_ch0), ST9/1(In)
  [MONIT_POS_Q] -> TDM_monit_pos_1/4(din_ch2)
  Reinterpret/1 -> TDM_monit_pos_1/5(din_ch3)
  [MONIT_POS_SUM] -> Reinterpret/1
  TDM_monit_pos_1/1(dout) -> monit_pos_1/1(din), ST10/1(In)
  TDM_monit_pos_1/2(ch_out) -> monit_pos_1/2(ch_in)
  Constant11/1 -> TDM_monit_pos_1/1(rst), ST7/1(In)
  [Kx] -> Kx_monit_mult1/2(In2)
  [Kx] -> Kx_q_monit_mult1/2(In2)
  [Ksum] -> Ksum_tbt_mult1/2(In2)
  [Ky] -> Kx_q_fofb_mult2/2(In2)
  monit_pos_1/1(monit_1_pos_x) -> Kx_monit_mult1/1(In1)
  Kx_monit_mult1/1(Out1) -> x_monit_1_o/1
  Kx_q_fofb_mult2/1(Out1) -> y_monit_1_o/1
  monit_pos_1/2(monit_1_pos_y) -> Kx_q_fofb_mult2/1(In1)
  monit_pos_1/3(monit_1_pos_q) -> Kx_q_monit_mult1/1(In1)
  monit_pos_1/4(monit_1_sum) -> Ksum_tbt_mult1/1(In1)
  Kx_q_monit_mult1/1(Out1) -> q_monit_1_o/1
  Ksum_tbt_mult1/1(Out1) -> sum_monit_1_o/1

== system ddc_bpm_476_066/ADC_16bit_ch0 ==
  A : Inport  OutDataTypeStr=double
  Conversion3 : DataTypeConversion  OutDataTypeStr=fixdt(1,16,2/2^16/1,0/1)  ConvertRealWorld=Stored Integer (SI)  LockScale=on
  Quantizer : Quantizer  QuantizationInterval=1  SampleTime=dt_sim
  Sampler : ZeroOrderHold  SampleTime=1/Fs_adc
  Saturation : Saturate  UpperLimit=65536/2-1  LowerLimit=-65536/2  OutDataTypeStr=Inherit: Inherit via back propagation
  scale : Gain  Gain=2^16/2  SaturateOnIntegerOverflow=on  OutDataTypeStr=Inherit: Same as input  ParamDataTypeStr=Inherit: Same as input
  D : Outport
  wires:
  A/1 -> scale/1
  Conversion3/1 -> D/1
  Quantizer/1 -> Saturation/1
  Sampler/1 -> Quantizer/1
  Saturation/1 -> Conversion3/1
  scale/1 -> Sampler/1

== system ddc_bpm_476_066/ADC_16bit_ch1 ==
  A : Inport  OutDataTypeStr=double
  Conversion3 : DataTypeConversion  OutDataTypeStr=fixdt(1,16,2/2^16/1,0/1)  ConvertRealWorld=Stored Integer (SI)  LockScale=on
  Quantizer : Quantizer  QuantizationInterval=1  SampleTime=dt_sim
  Sampler : ZeroOrderHold  SampleTime=1/Fs_adc
  Saturation : Saturate  UpperLimit=65536/2-1  LowerLimit=-65536/2  OutDataTypeStr=Inherit: Inherit via back propagation
  scale : Gain  Gain=2^16/2  SaturateOnIntegerOverflow=on  OutDataTypeStr=Inherit: Same as input  ParamDataTypeStr=Inherit: Same as input
  D : Outport
  wires:
  A/1 -> scale/1
  Conversion3/1 -> D/1
  Quantizer/1 -> Saturation/1
  Sampler/1 -> Quantizer/1
  Saturation/1 -> Conversion3/1
  scale/1 -> Sampler/1

== system ddc_bpm_476_066/ADC_16bit_ch2 ==
  A : Inport  OutDataTypeStr=double
  Conversion3 : DataTypeConversion  OutDataTypeStr=fixdt(1,16,2/2^16/1,0/1)  ConvertRealWorld=Stored Integer (SI)  LockScale=on
  Quantizer : Quantizer  QuantizationInterval=1  SampleTime=dt_sim
  Sampler : ZeroOrderHold  SampleTime=1/Fs_adc
  Saturation : Saturate  UpperLimit=65536/2-1  LowerLimit=-65536/2  OutDataTypeStr=Inherit: Inherit via back propagation
  scale : Gain  Gain=2^16/2  SaturateOnIntegerOverflow=on  OutDataTypeStr=Inherit: Same as input  ParamDataTypeStr=Inherit: Same as input
  D : Outport
  wires:
  A/1 -> scale/1
  Conversion3/1 -> D/1
  Quantizer/1 -> Saturation/1
  Sampler/1 -> Quantizer/1
  Saturation/1 -> Conversion3/1
  scale/1 -> Sampler/1

== system ddc_bpm_476_066/ADC_16bit_ch3 ==
  A : Inport  OutDataTypeStr=double
  Conversion3 : DataTypeConversion  OutDataTypeStr=fixdt(1,16,2/2^16/1,0/1)  ConvertRealWorld=Stored Integer (SI)  LockScale=on
  Quantizer : Quantizer  QuantizationInterval=1  SampleTime=dt_sim
  Sampler : ZeroOrderHold  SampleTime=1/Fs_adc
  Saturation : Saturate  UpperLimit=65536/2-1  LowerLimit=-65536/2  OutDataTypeStr=Inherit: Inherit via back propagation
  scale : Gain  Gain=2^16/2  SaturateOnIntegerOverflow=on  OutDataTypeStr=Inherit: Same as input  ParamDataTypeStr=Inherit: Same as input
  D : Outport
  wires:
  A/1 -> scale/1
  Conversion3/1 -> D/1
  Quantizer/1 -> Saturation/1
  Sampler/1 -> Quantizer/1
  Saturation/1 -> Conversion3/1
  scale/1 -> Sampler/1

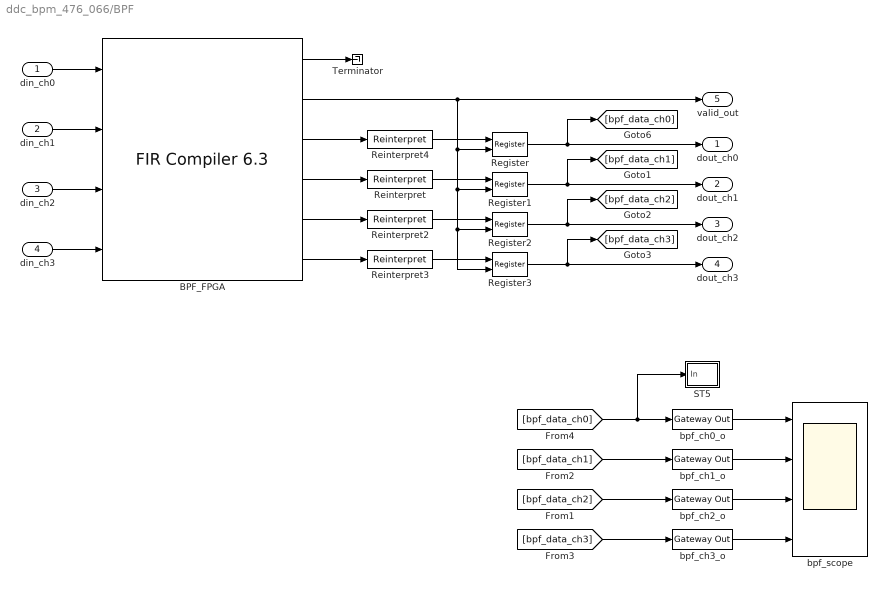
== system ddc_bpm_476_066/BPF ==
  din_ch0 : Inport
  din_ch1 : Inport  Port=2
  din_ch2 : Inport  Port=3
  din_ch3 : Inport  Port=4
  BPF_FPGA : xbsIndex_r4/FIR Compiler 6.3   coefficientvector=Hbpf_adc.Numerator  coefficient_sets=1  coefficient_reload=off  filter_type=Single_Rate  rate_change_type=Integer  interpolation_rate=1  decimation_rate=1  zero_pack_factor=1  channel_sequence=Basic  number_channels=1  pattern_list='P4-0,P4-1,P4-2,P4-3,P4-4'  number_paths=4  ratespecification=Hardware_Oversampling_Rate  sampleperiod=2  hardwareoversamplingrate=n_ovs  coefficient_sign=Signed  quantization=Quantize_Only  coefficient_width=16  bestprecision=on  coefficient_fractional_bits=17  coefficient_structure=Inferred  output_rounding_mode=Convergent_Rounding_to_Even  output_width=24  filter_architecture=Systolic_Multiply_Accumulate  optimization_goal=Area  data_buffer_type=Automatic  coefficient_buffer_type=Automatic  input_buffer_type=Automatic  output_buffer_type=Automatic  preference_for_other_storage=Automatic  multi_column_support=Automatic  columnconfig='10'  inter_column_pipe_length=4  data_has_tlast=Not_Required  m_data_has_tready=off  s_data_has_fifo=off  s_data_has_tuser=Not_Required  m_data_has_tuser=Not_Required  s_config_sync_mode=On_Vector  s_config_method=Single  num_reload_slots=1  has_aclken=off  has_aresetn=off  infoeditControl=ARESETn must be asserted for a minmum of 2 cycles  trim_axipin_name=on  passband_min=0.0  passband_max=0.5  stopband_min=0.5  stopband_max=1.0  filter_selection=1  gui_behaviour=Sysgen_GUI  data_sign=Signed  data_width=16  data_fractional_bits=0  data_tuser_width=1  wrapper_available=true  ip_wrap_arbitrary_binary_point=true  simulation_type=external_xfix  simulation_model=firv6_3_CModel:firv6_3_cmodel  ip_name=FIR Compiler  ip_version=6.3  dsptool_ready=true  ipcore_usecache=true  ipcore_useipmodelcache=true  ipcore_xco_need_fpga_part=true  port_translation_map={ 'aclken' => 'en', 'aresetn' => 'rst' }  run_core_at_system_period=true  ipcore_fpga_part=xlipgetpartsetting(gcb, {'virtex6', 'xc6vlx75t', '-3', 'ff784'})  block_type=fir_compiler_v6_3
      settings: infoedit=Maximum Possible : Maximizes oversampling rate. Abstracted input handshake (no s_data_tvalid) and automatic rate propagation.<br>Hardware Oversampling Rate : Specifies oversampling rate relative to the input sample period. Abstracted input handshake (no s_data_tvalid) and automatic rate propagation.<br>Sample Period : Specifies absolute oversampling rate. No input handshake abstraction (exposes s_data_tvalid) and no rate propagation.
  Register{,1..3} (4 alike) : xbsIndex_r4/Register  init=0  rst=off  en=on  dbl_ovrd=off  block_type=register
  Reinterpret{,2..4} (4 alike) : xbsIndex_r4/Reinterpret  force_arith_type=off  arith_type=Unsigned  force_bin_pt=on  bin_pt=22  block_type=reinterpret
  ST5 : Subsystem
  Terminator : Terminator
  bpf_ch0_o : xbsIndex_r4/Gateway Out  inherit_from_input=on  hdl_port=on  timing_constraint=Data Rate  locs_specified=off  LOCs={}  UseAsDAC=off  DACChannel='1'  block_type=gatewayout
      settings: infoedit="Gateway out block.  Converts Xilinx fixed-point or floating-point type inputs into ouputs of type Simulink integer, single, double, or fixed point.<br><br>Hardware notes:  In hardware these blocks become top level output ports or are discarded, depending on how they are configured."
  bpf_ch1_o : xbsIndex_r4/Gateway Out  inherit_from_input=on  hdl_port=on  timing_constraint=Data Rate  locs_specified=off  LOCs={}  UseAsDAC=off  DACChannel='1'  block_type=gatewayout
      settings: infoedit="Gateway out block.  Converts Xilinx fixed-point or floating-point type inputs into ouputs of type Simulink integer, single, double, or fixed point.<br><br>Hardware notes:  In hardware these blocks become top level output ports or are discarded, depending on how they are configured."
  bpf_ch2_o : xbsIndex_r4/Gateway Out  inherit_from_input=on  hdl_port=on  timing_constraint=Data Rate  locs_specified=off  LOCs={}  UseAsDAC=off  DACChannel='1'  block_type=gatewayout
      settings: infoedit="Gateway out block.  Converts Xilinx fixed-point or floating-point type inputs into ouputs of type Simulink integer, single, double, or fixed point.<br><br>Hardware notes:  In hardware these blocks become top level output ports or are discarded, depending on how they are configured."
  bpf_ch3_o : xbsIndex_r4/Gateway Out  inherit_from_input=on  hdl_port=on  timing_constraint=Data Rate  locs_specified=off  LOCs={}  UseAsDAC=off  DACChannel='1'  block_type=gatewayout
      settings: infoedit="Gateway out block.  Converts Xilinx fixed-point or floating-point type inputs into ouputs of type Simulink integer, single, double, or fixed point.<br><br>Hardware notes:  In hardware these blocks become top level output ports or are discarded, depending on how they are configured."
  bpf_scope : Scope  NumInputPorts=4
      settings: TimeRange=0.00011214  YMin=-0.1~-1.5~-0.002~-1.5  YMax=1~1.5~0.00075~1.5  SaveName=ScopeData16  MaxDataPoints=1000000  SampleInput=on
  dout_ch0 : Outport
  dout_ch1 : Outport  Port=2
  dout_ch2 : Outport  Port=3
  dout_ch3 : Outport  Port=4
  valid_out : Outport  Port=5
  wires:
  din_ch0/1 -> BPF_FPGA/1
  BPF_FPGA/1 -> Terminator/1
  BPF_FPGA/2 -> valid_out/1, Register/2, Register1/2, Register2/2, Register3/2
  BPF_FPGA/3 -> Reinterpret4/1
  BPF_FPGA/5 -> Reinterpret2/1
  din_ch1/1 -> BPF_FPGA/2
  BPF_FPGA/4 -> Reinterpret/1
  bpf_ch3_o/1 -> bpf_scope/4
  bpf_ch2_o/1 -> bpf_scope/3
  bpf_ch1_o/1 -> bpf_scope/2
  bpf_ch0_o/1 -> bpf_scope/1
  din_ch2/1 -> BPF_FPGA/3
  din_ch3/1 -> BPF_FPGA/4
  BPF_FPGA/6 -> Reinterpret3/1
  [bpf_data_ch0] -> bpf_ch0_o/1, ST5/1(In)
  [bpf_data_ch1] -> bpf_ch1_o/1
  [bpf_data_ch3] -> bpf_ch3_o/1
  [bpf_data_ch2] -> bpf_ch2_o/1
  Register/1 -> dout_ch0/1, [bpf_data_ch0]
  Register1/1 -> dout_ch1/1, [bpf_data_ch1]
  Reinterpret4/1 -> Register/1
  Reinterpret/1 -> Register1/1
  Reinterpret2/1 -> Register2/1
  Reinterpret3/1 -> Register3/1
  Register2/1 -> dout_ch2/1, [bpf_data_ch2]
  Register3/1 -> dout_ch3/1, [bpf_data_ch3]

== system ddc_bpm_476_066/FOFB_amp ==
  Q_in0 : Inport
  I_in0 : Inport  Port=2
  ch_in0 : Inport  Port=3
  Q_in1 : Inport  Port=4
  I_in1 : Inport  Port=5
  ch_in1 : Inport  Port=6
  ST1 : Subsystem
  ST5 : Subsystem
  TDDM_fofb_amp_4ch : Subsystem
  Terminator{,1..3} (4 alike) : Terminator
  fofb_amp0 : Subsystem
  fofb_amp1 : Subsystem
  amp_out0 : Outport
  amp_out1 : Outport  Port=2
  amp_out2 : Outport  Port=3
  amp_out3 : Outport  Port=4
  wires:
  Q_in0/1 -> fofb_amp0/1(Q_in)
  I_in0/1 -> fofb_amp0/2(I_in)
  ch_in0/1 -> fofb_amp0/3(ch_in)
  Q_in1/1 -> fofb_amp1/1(Q_in)
  I_in1/1 -> fofb_amp1/2(I_in)
  ch_in1/1 -> fofb_amp1/3(ch_in)
  TDDM_fofb_amp_4ch/1(amp_out0) -> amp_out0/1, ST1/1(In)
  TDDM_fofb_amp_4ch/2(amp_out1) -> amp_out1/1
  TDDM_fofb_amp_4ch/3(amp_out2) -> amp_out2/1
  TDDM_fofb_amp_4ch/4(amp_out3) -> amp_out3/1
  fofb_amp0/1(amp_out) -> TDDM_fofb_amp_4ch/1(amp_in0), ST5/1(In)
  fofb_amp0/4(ch_out) -> TDDM_fofb_amp_4ch/2(ch_in0)
  fofb_amp1/1(amp_out) -> TDDM_fofb_amp_4ch/3(amp_in1)
  fofb_amp1/4(ch_out) -> TDDM_fofb_amp_4ch/4(ch_in1)
  fofb_amp0/2(phase_out) -> Terminator/1
  fofb_amp0/3(valid_out) -> Terminator1/1
  fofb_amp1/2(phase_out) -> Terminator2/1
  fofb_amp1/3(valid_out) -> Terminator3/1

== system ddc_bpm_476_066/Ksum_fofb_mult ==
  In1 : Inport
  In2 : Inport  Port=2
  Cast_truncate1 : Subsystem
  Kx_tbt : xbsIndex_r4/Mult  precision=Full  arith_type="Signed  (2's comp)"  n_bits=16  bin_pt=14  quantization=Truncate  overflow=Wrap  en=off  latency=8  dbl_ovrd=off  use_behavioral_HDL=off  opt=Speed  use_embedded=off  optimum_pipeline=on  pipeline=on  use_rpm=on  placement_style=Triangular  block_type=mult
  Register : xbsIndex_r4/Register  init=0  rst=off  en=off  dbl_ovrd=off  block_type=register
  Out1 : Outport
  wires:
  Kx_tbt/1 -> Cast_truncate1/1(In1)
  In1/1 -> Kx_tbt/1
  Cast_truncate1/1(Out1) -> Register/1
  In2/1 -> Kx_tbt/2
  Register/1 -> Out1/1

== system ddc_bpm_476_066/Ksum_tbt_mult1 ==
  In1 : Inport
  In2 : Inport  Port=2
  Cast_truncate1 : Subsystem
  Kx_tbt : xbsIndex_r4/Mult  precision=Full  arith_type="Signed  (2's comp)"  n_bits=16  bin_pt=14  quantization=Truncate  overflow=Wrap  en=off  latency=8  dbl_ovrd=off  use_behavioral_HDL=off  opt=Speed  use_embedded=off  optimum_pipeline=on  pipeline=on  use_rpm=on  placement_style=Triangular  block_type=mult
  Register : xbsIndex_r4/Register  init=0  rst=off  en=off  dbl_ovrd=off  block_type=register
  Out1 : Outport
  wires:
  Kx_tbt/1 -> Cast_truncate1/1(In1)
  In1/1 -> Kx_tbt/1
  Cast_truncate1/1(Out1) -> Register/1
  In2/1 -> Kx_tbt/2
  Register/1 -> Out1/1
